simulink model "Inner_and_Outer_Loop_Graph"  (R2013a)
settings: Solver=ode45  StartTime=0.0  StopTime=10.0  RelTol=1e-3
settings Model: Creator=Administrator  LastModifiedBy=Administrator

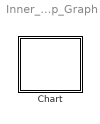
== system Inner_and_Outer_Loop_Graph ==
  Chart : Stateflow chart  TreatAsAtomicUnit=on

== stateflow chart Inner_and_Outer_Loop_Graph/Chart ==
  note: Z
  state Outer  Loop [group]
    Control
  state Inner Loop [group]
    Control
  state Quadrotor [group]
    System
  state Observer [group]
  Outer  Loop -> Inner Loop : V1
  (junction 31) -> Outer  Loop : Zd, Z'd
  Inner Loop -> Quadrotor : U1
  Quadrotor -> (junction 19)
  (junction 19) -> Inner Loop [order 1] : Phi ,Theta
  (junction 19) -> Observer [order 2] : z, Phi
      |
      |  Theta
  Observer -> Outer  Loop : estZ,estZ'
